simulink model "Pulse_timer_N_square"  (R2015a)
settings: Solver=ode23t  StartTime=0.0  StopTime=1e-3  RelTol=1e-3
libraries: fl_lib x16, elec_lib x9, nesl_utility x6
settings Model: Creator=saifur  LastModifiedBy=saifur
settings DebuggingCC: UnconnectedInputMsg=none  UnconnectedOutputMsg=none  UnconnectedLineMsg=none

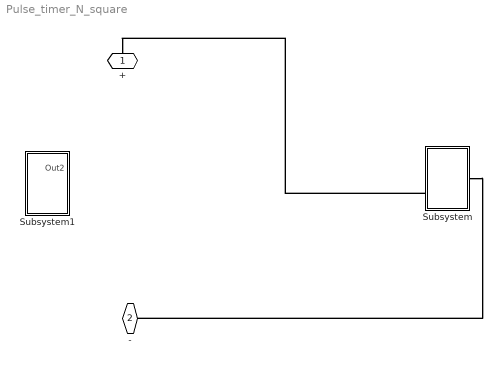
== system Pulse_timer_N_square ==
  Subsystem : Subsystem
  Subsystem1 : Subsystem
  + : PMIOPort  Port=1  Side=Left
  - : PMIOPort  Port=2  Side=Right
  connections:
  +/RConn1 -- ?
  -/RConn1 -- ?

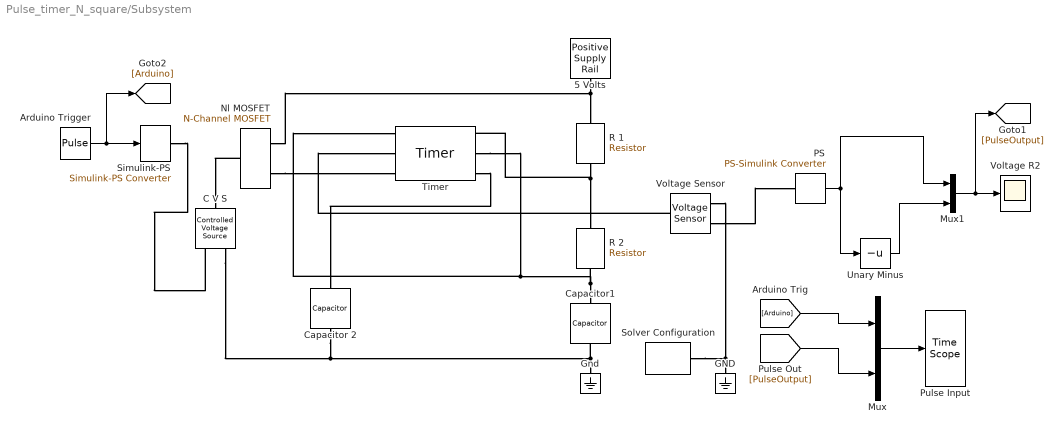
== system Pulse_timer_N_square/Subsystem ==
  5 Volts : elec_lib/Sources/Positive Supply Rail  v0=5 V
  Arduino Trigger : DiscretePulseGenerator  PulseType=Time based  Amplitude=5  Period=0.0001  PulseWidth=50
  C V S : fl_lib/Electrical/Electrical Sources/Controlled Voltage Source
  Capacitor 2 : fl_lib/Electrical/Electrical Elements/Capacitor  c=0.01 uF  r=1e-6 Ohm  g=0 1/Ohm  i_specify=off  i_priority=High  i=0 A  v_specify=off  v_priority=High  v=0 V  vc_specify=off  vc_priority=High  vc=0 V
  Capacitor1 : fl_lib/Electrical/Electrical Elements/Capacitor  c=0.47 nF  r=1e-6 Ohm  g=0 1/Ohm  i_specify=off  i_priority=High  i=0 A  v_specify=off  v_priority=High  v=0 V  vc_specify=off  vc_priority=High  vc=0 V
  GND : fl_lib/Electrical/Electrical Elements/Electrical Reference
  Gnd : fl_lib/Electrical/Electrical Elements/Electrical Reference
  Mux : Mux  Inputs=2
  Mux1 : Mux  Inputs=2
  Nl MOSFET : elec_lib/Semiconductor Devices/N-Channel MOSFET  parameterization=1  prmDatasheet=1  prmEquCoeff=1  Beta=5 A/V^2  Rds=0.025 Ohm  Id=6 A  Vgs=10 V  Vth=1.7 V  lam=0 1/V  Tmeas=25 C  RS=1e-4 Ohm  RD=0.01 Ohm  C_param=1  C_GS=270 pF  C_GD=80 pF  C_iss=350 pF  C_rss=80 pF  C_oss=0 pF  C_GS_vec=[ 270 300 290 280 295 255 ] pF  C_GD_vec=[ 450 400 300 190 95 55 ] pF  C_iss_vec=[ 720 700 590 470 390 310 ] pF  C_rss_vec=[ 450 400 300 190 95 55 ] pF  C_oss_vec=[ 900 810 690 420 270 170 ] pF  C_Vds_vec=[ 0.1 0.3 1 3 10 30 ] V  charge_linearity_param=1  C_OX=200 pF  V_C_OX=-0.5 V  dVth_dT=-6 mV/K  Rds_T2=0.037 Ohm  Tmeas2=125 C  BEXDatasheet=-1.5  BEXEquCoeff=-1.5  TdeviceDatasheet=25 C  TdeviceEquCoeff=25 C  Rth=[ 0 10 ] K/W  thermal_mass_parameterization=1  thermal_mass=[ 0 1 ] J/K  thermal_time_constant=[ 0 10 ] s  thermal_mass_initial_temperatures=[ 25 25 ] C
  PS : nesl_utility/PS-Simulink Converter  PhysicalDomain=network_engine_domain  SubClassName=ps_output  LeftPortType=input  RightPortType=output  PseudoPeriodic=off  Frequencies=[]  Unit=1  AffineConversion=off
  Pulse Input : TimeScope
  R 1 : elec_lib/Passive Devices/Resistor  R=1 kOhm  noise_mode=0  Tdevice=25 C  sample_time=0.001 s  repeatability=1  auto_seed=545404223  user_seed=0
  R 2 : elec_lib/Passive Devices/Resistor  R=3.5 kOhm  noise_mode=0  Tdevice=25 C  sample_time=0.001 s  repeatability=1  auto_seed=2715962282  user_seed=0
  "Simulink-PS " : nesl_utility/Simulink-PS Converter  PhysicalDomain=network_engine_domain  SubClassName=ps_input  LeftPortType=input  RightPortType=output  PseudoPeriodic=off  Frequencies=[]  NoiseDistribution=none  NoiseParameters=[]  Unit=V  AffineConversion=off  InputFiltering=off  SimscapeFilterOrder=1  InputFilterTimeConstant=0.001  UdotUserProvided=1
  Solver Configuration : nesl_utility/Solver Configuration  PhysicalDomain=network_engine_domain  SubClassName=solver  LeftPortType=input  RightPortType=generic  Accelerate=off  Tones=[]  Harmonics=[]  SimulateNoise=off  Profile=off  UseLocalSampling=off  EnableSwitchedLinearOptims=on  FrequencyDomain=off  UseCCode=off  RelTol=0.001  AbsTol=1e-06  MinStep=1e-09  ToWorkspace=off  RevertToSquareIcSolve=off  NumHomotopyIterations=100  DoDC=off  ResidualTolerance=1e-09  UseLocalSolver=off  LocalSolverChoice=NE_TRAPEZOIDAL_ADVANCER  LocalSolverSampleTime=0.001  DoFixedCost=off  MaxNonlinIter=3  MaxModeIter=2  LinearAlgebra=Full  DelaysMemoryBudget=1024  AutomaticFiltering=on  FilteringTimeConstant=0.001
  Timer : elec_lib/Integrated Circuits/Timer  V_CC=5 V  V_OL=0 V  V_OH=5 V  R_OUT=8 Ohm  Delay=1e-7 s  R_DIV=5 kOhm  R_closed=12 Ohm  R_open=5e+8 Ohm
  Unary Minus : UnaryMinus
  Voltage R2 : Scope
      settings: YMin=-5.5  YMax=5.5  SaveName=ScopeData3  Decimation=2
  Voltage Sensor : fl_lib/Electrical/Electrical Sensors/Voltage Sensor
  wires:
  PS/1 -> Unary Minus/1, Mux1/1
  Unary Minus/1 -> Mux1/2
  Arduino Trigger/1 -> "Simulink-PS "/1, [Arduino]
  [Arduino] -> Mux/1
  [PulseOutput] -> Mux/2
  Mux/1 -> Pulse Input/1
  Mux1/1 -> [PulseOutput], Voltage R2/1
  connections:
  R 1/RConn1 -- Timer/RConn1 -- R 2/LConn1
  Timer/RConn3 -- Capacitor 2/LConn1
  Capacitor 2/RConn1 -- Gnd/LConn1 -- Capacitor1/RConn1 -- C V S/RConn2
  5 Volts/RConn1 -- Nl MOSFET/RConn1 -- R 1/LConn1
  Timer/RConn2 -- R 2/RConn1 -- Capacitor1/LConn1 -- Timer/LConn1
  Voltage Sensor/RConn1 -- PS/LConn1
  Voltage Sensor/LConn1 -- Timer/LConn2
  Voltage Sensor/RConn2 -- Solver Configuration/RConn1 -- GND/LConn1
  Nl MOSFET/RConn2 -- Timer/LConn3
  Nl MOSFET/LConn1 -- C V S/LConn1
  "Simulink-PS "/RConn1 -- C V S/RConn1

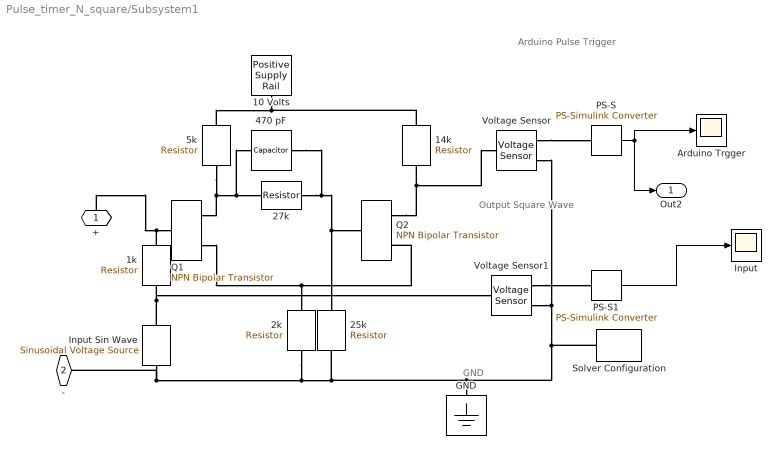
== system Pulse_timer_N_square/Subsystem1 ==
  note: Output Square Wave
  note: GND
  note: Arduino Pulse Trigger
  10 Volts : elec_lib/Sources/Positive Supply Rail  v0=10 V
  14k : fl_lib/Electrical/Electrical Elements/Resistor  R=14 kOhm  i_specify=off  i_priority=High  i=0 A  v_specify=off  v_priority=High  v=0 V
  1k : fl_lib/Electrical/Electrical Elements/Resistor  R=1 kOhm  i_specify=off  i_priority=High  i=0 A  v_specify=off  v_priority=High  v=0 V
  25k : fl_lib/Electrical/Electrical Elements/Resistor  R=25 kOhm  i_specify=off  i_priority=High  i=0 A  v_specify=off  v_priority=High  v=0 V
  27k : fl_lib/Electrical/Electrical Elements/Resistor  R=27 kOhm  i_specify=off  i_priority=High  i=0 A  v_specify=off  v_priority=High  v=0 V
  2k : fl_lib/Electrical/Electrical Elements/Resistor  R=2 kOhm  i_specify=off  i_priority=High  i=0 A  v_specify=off  v_priority=High  v=0 V
  470 pF : fl_lib/Electrical/Electrical Elements/Capacitor  c=470 pF  r=1e-06 Ohm  g=0 1/Ohm  i_specify=off  i_priority=High  i=0 A  v_specify=off  v_priority=High  v=0 V  vc_specify=on  vc_priority=High  vc=0 V
  5k : fl_lib/Electrical/Electrical Elements/Resistor  R=5 kOhm  i_specify=off  i_priority=High  i=0 A  v_specify=off  v_priority=High  v=0 V
  Arduino Trgger : Scope
      settings: TimeRange=0.1  YMin=0  YMax=15
  GND : fl_lib/Electrical/Electrical Elements/Electrical Reference
  Input : Scope
      settings: TimeRange=0.1
  Input Sin Wave : elec_lib/Additional Components/SPICE-Compatible Components/Sources/Sinusoidal Voltage Source  VO=0 V  VA=5 V  FREQ=50 Hz  TD=0 s  DF=0 1/s  OMEGA=0 rad/s
  PS-S : nesl_utility/PS-Simulink Converter  PhysicalDomain=network_engine_domain  SubClassName=ps_output  LeftPortType=input  RightPortType=output  PseudoPeriodic=off  Frequencies=[]  Unit=1  AffineConversion=off
  PS-S1 : nesl_utility/PS-Simulink Converter  PhysicalDomain=network_engine_domain  SubClassName=ps_output  LeftPortType=input  RightPortType=output  PseudoPeriodic=off  Frequencies=[]  Unit=1  AffineConversion=off
  Q1 : elec_lib/Semiconductor Devices/NPN Bipolar Transistor  parameterization=1  prmDatasheet=1  prmEquCoeff=1  BF=100  IS=1e-14 A  ec=1  VAF=200 V  hfe=100  hoe=5e-05 1/Ohm  Ic_h=1 mA  Vce_h=5 V  V1=0.55 V  I1=0.5 mA  BR=1  Tmeas=25 C  RC=0.1 Ohm  RE=0.1 Ohm  RB=0.1 Ohm  C_BC=5 pF  C_BE=5 pF  TF=0 us  TR=0 us  hfe_T2=125  XTB=0  V1_T2=0.45 V  I1_T2=0.5 mA  Tmeas2=125 C  EG=1.11 eV  XTI=3  TdeviceDatasheet=25 C  TdeviceEquCoeff=25 C  Rth=[ 0 10 ] K/W  thermal_mass_parameterization=1  thermal_mass=[ 0 1 ] J/K  thermal_time_constant=[ 0 10 ] s  thermal_mass_initial_temperatures=[ 25 25 ] C
  Q2 : elec_lib/Semiconductor Devices/NPN Bipolar Transistor  parameterization=1  prmDatasheet=1  prmEquCoeff=1  BF=100  IS=1e-14 A  ec=1  VAF=200 V  hfe=100  hoe=5e-05 1/Ohm  Ic_h=1 mA  Vce_h=5 V  V1=0.55 V  I1=0.5 mA  BR=1  Tmeas=25 C  RC=0.1 Ohm  RE=0.1 Ohm  RB=0.1 Ohm  C_BC=5 pF  C_BE=5 pF  TF=0 us  TR=0 us  hfe_T2=125  XTB=0  V1_T2=0.45 V  I1_T2=0.5 mA  Tmeas2=125 C  EG=1.11 eV  XTI=3  TdeviceDatasheet=25 C  TdeviceEquCoeff=25 C  Rth=[ 0 10 ] K/W  thermal_mass_parameterization=1  thermal_mass=[ 0 1 ] J/K  thermal_time_constant=[ 0 10 ] s  thermal_mass_initial_temperatures=[ 25 25 ] C
  Solver Configuration : nesl_utility/Solver Configuration  PhysicalDomain=network_engine_domain  SubClassName=solver  LeftPortType=input  RightPortType=generic  Accelerate=off  Tones=[]  Harmonics=[]  SimulateNoise=off  Profile=off  UseLocalSampling=off  EnableSwitchedLinearOptims=on  FrequencyDomain=off  UseCCode=off  RelTol=0.001  AbsTol=1e-06  MinStep=1e-09  ToWorkspace=off  RevertToSquareIcSolve=off  NumHomotopyIterations=100  DoDC=off  ResidualTolerance=1e-9  UseLocalSolver=off  LocalSolverChoice=NE_BACKWARD_EULER_ADVANCER  LocalSolverSampleTime=0.001  DoFixedCost=off  MaxNonlinIter=12  MaxModeIter=2  LinearAlgebra=Sparse  DelaysMemoryBudget=1024  AutomaticFiltering=on  FilteringTimeConstant=0.001
  Voltage Sensor : fl_lib/Electrical/Electrical Sensors/Voltage Sensor
  Voltage Sensor1 : fl_lib/Electrical/Electrical Sensors/Voltage Sensor
  + : PMIOPort  Port=1  Side=Left
  - : PMIOPort  Port=2  Side=Right
  Out2 : Outport
  wires:
  PS-S1/1 -> Input/1
  PS-S/1 -> Out2/1, Arduino Trgger/1
  connections:
  5k/RConn1 -- Q1/RConn1 -- 27k/RConn1 -- 470 pF/LConn1
  Q1/RConn2 -- Q2/RConn2 -- 2k/LConn1
  Input Sin Wave/LConn1 -- 1k/RConn1 -- Voltage Sensor1/LConn1
  Voltage Sensor/RConn1 -- PS-S/LConn1
  Q1/LConn1 -- 1k/LConn1 -- +/RConn1
  Q2/RConn1 -- 14k/RConn1 -- Voltage Sensor/LConn1
  14k/LConn1 -- 10 Volts/RConn1 -- 5k/LConn1
  27k/LConn1 -- Q2/LConn1 -- 25k/LConn1 -- 470 pF/RConn1
  Voltage Sensor1/RConn1 -- PS-S1/LConn1
  2k/RConn1 -- Voltage Sensor/RConn2 -- Voltage Sensor1/RConn2 -- Solver Configuration/RConn1 -- GND/LConn1 -- 25k/RConn1 -- Input Sin Wave/RConn1 -- -/RConn1
